simulink model "Code_for_Chp4_2DoF_LiteOfAllPlus"  (R2016b)
settings: Solver=ode4  StartTime=0  StopTime=30  FixedStep=0.0005  MaxStep=0.005  MinStep=0.001  RelTol=0.5
libraries: dspindex x2
settings Model: ExtModeTrigMode=oneshot  ExtModeArmWhenConnect=off  Creator=hp  LastModifiedBy=sfijdl
settings DataIOCC: ExternalInput=untitled.getElement(1),[],[],[],[],[],[],[],[],[],[],[],[],[],[],[],[],[],[]  SaveFormat=Array  SignalLoggingSaveFormat=ModelDataLogs  SignalLoggingName=sigsOut
settings OptimizationCC: DefaultParameterBehavior=Inlined  UseDivisionForNetSlopeComputation=on  UseFloatMulNetSlope=on  InlineInvariantSignals=on  PassReuseOutputArgsAs=Individual arguments  ExpressionDepthLimit=2147483647  ZeroExternalMemoryAtStartup=off  ZeroInternalMemoryAtStartup=off  NoFixptDivByZeroProtection=on  EfficientFloat2IntCast=on  LifeSpan=1
settings DebuggingCC: SaveWithParameterizedLinksMsg=none  UnderspecifiedInitializationDetection=Classic  MergeDetectMultiDrivingBlocksExec=none  SignalResolutionControl=TryResolveAllWithWarning  MultiTaskDSMMsg=warning  MultiTaskCondExecSysMsg=none  MultiTaskRateTransMsg=warning  ParameterTunabilityLossMsg=error  FcnCallInpInsideContextMsg=warning  StateNameClashWarn=warning  SFUnexpectedBacktrackingDiag=warning  SFNoUnconditionalDefaultTransitionDiag=warning  SFExecutionAtInitializationDiag=none
settings HardwareCC: TargetBitPerPointer=64  TargetBitPerSizeT=64  TargetBitPerPtrDiffT=64  TargetLongLongMode=on  TargetIntDivRoundTo=Zero  TargetEndianess=LittleEndian  TargetWordSize=64  TargetHWDeviceType=MATLAB Host  ProdEqTarget=off
settings ModelReferenceCC: PropagateSignalLabelsOutOfModel=off
settings RTWCC: SystemTargetFile=ert.tlc  TemplateMakefile=ert_default_tmf  Description=Embedded Coder  GenerateReport=on  IncludeHyperlinkInReport=on  LaunchReport=on  GenerateTraceInfo=on  GenerateTraceReport=on  GenerateTraceReportSl=on  GenerateTraceReportSf=on  GenerateTraceReportEml=on  GenerateCodeMetricsReport=on
settings CodeAppCC: ForceParamTrailComments=on  IgnoreCustomStorageClasses=off  MaxIdLength=128  OperatorAnnotations=on  SimulinkDataObjDesc=on  SFDataObjDesc=on  MATLABFcnDesc=on  CustomSymbolStrGlobalVar=rt$N$M  CustomSymbolStrType=$N$M  CustomSymbolStrFcn=$N$M$F  CustomSymbolStrMacro=$N$M  InsertBlockDesc=on  MATLABSourceComments=on
settings ERTTargetCC: GenerateSampleERTMain=on  CombineSignalStateStructs=on  SupportComplex=off  SupportNonInlinedSFcns=on  InlinedParameterPlacement=NonHierarchical  ERTCustomFileTemplate=example_file_process.tlc  ERTFilePackagingFormat=CompactWithDataFile
settings ConfigComp: CovMetricSettings=dw  CovHtmlReporting=on  CovSaveCumulativeToWorkspaceVar=on  CovSaveSingleToWorkspaceVar=on  CovExternalEMLEnable=off

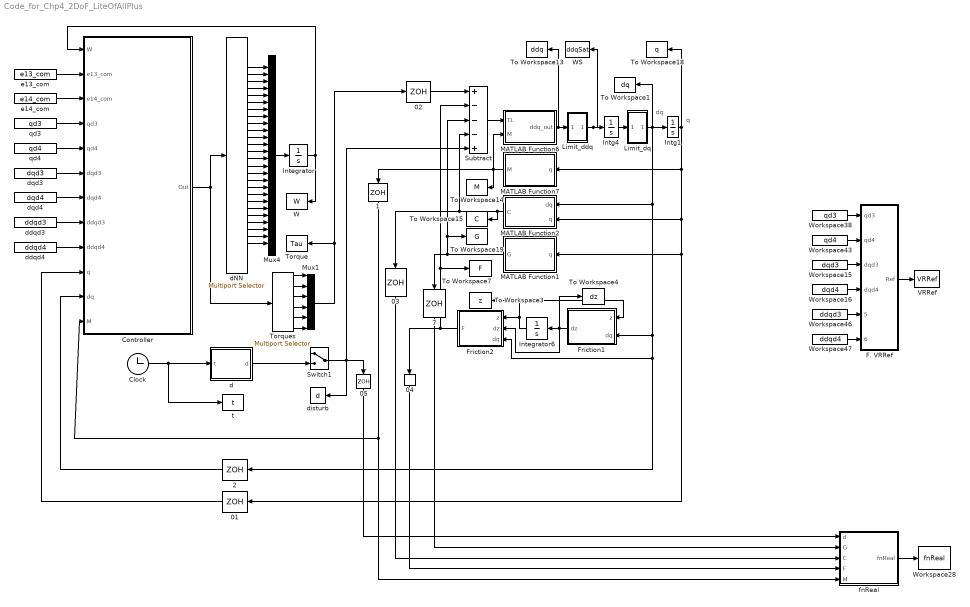
== system Code_for_Chp4_2DoF_LiteOfAllPlus ==
  note: q
  note: dq
  01 : ZeroOrderHold  SampleTime=0.0025
  02 : ZeroOrderHold  SampleTime=0.0025
  03 : ZeroOrderHold  SampleTime=0.0025
  04 : ZeroOrderHold  SampleTime=0.0025
  05 : ZeroOrderHold  SampleTime=0.0025
  1 : ZeroOrderHold  SampleTime=0.0025
  2 : ZeroOrderHold  SampleTime=0.0025
  7 : ZeroOrderHold  SampleTime=0.0025
  Clock : Clock
  Controller : MATLAB Function  TreatAsAtomicUnit=on
  F. VRRef : MATLAB Function  TreatAsAtomicUnit=on
  Friction1 : MATLAB Function  TreatAsAtomicUnit=on
  Friction2 : MATLAB Function  TreatAsAtomicUnit=on
  Integrator : Integrator  InitialCondition=[zeros(2*13,1)]
  Integrator6 : Integrator  InitialCondition=[0;0;0;0;0;0]
  Intg1 : Integrator  InitialCondition=[0.005;-0.005]
  Intg4 : Integrator  InitialCondition=[-0.1705;0.1576]
  Limit_ddq : MATLAB Function  TreatAsAtomicUnit=on
  Limit_dq : MATLAB Function  TreatAsAtomicUnit=on
  MATLAB Function1 : MATLAB Function  TreatAsAtomicUnit=on
  MATLAB Function2 : MATLAB Function  TreatAsAtomicUnit=on
  MATLAB Function6 : MATLAB Function  TreatAsAtomicUnit=on
  MATLAB Function7 : MATLAB Function  TreatAsAtomicUnit=on
  Mux1 : Mux  Inputs=6
  Mux4 : Mux  Inputs=26
  Subtract : Sum  Inputs=+---+
  Switch1 : ManualSwitch
  To Workspace1 : ToWorkspace  VariableName=dq  SampleTime=-1
  To Workspace13 : ToWorkspace  VariableName=ddq  SampleTime=-1
  To Workspace14 : ToWorkspace  VariableName=M  SampleTime=-1
  To Workspace15 : ToWorkspace  VariableName=C  SampleTime=-1
  To Workspace18 : ToWorkspace  VariableName=q  SampleTime=-1
  To Workspace19 : ToWorkspace  VariableName=G  SampleTime=-1
  To Workspace3 : ToWorkspace  VariableName=z  SampleTime=-1
  To Workspace4 : ToWorkspace  VariableName=dz  SampleTime=-1
  To Workspace7 : ToWorkspace  VariableName=F  SampleTime=-1
  Torque : ToWorkspace  VariableName=Tau  SampleTime=-1
  Torques : dspindex/Multiport Selector  rowsOrCols=Rows  idxCellArray={27,28,29,30,31,32}  idxErrMode=Clip Index
  VRRef : ToWorkspace  VariableName=VRRef  SampleTime=-1
  W : ToWorkspace  VariableName=W  SampleTime=-1
  WS : ToWorkspace  VariableName=ddqSat  SampleTime=-1
  Workspace15 : FromWorkspace  VariableName=dqd3  SampleTime=0.0025  mask(DiscretizedSource){}
      mask init:
      | %zoh
  Workspace16 : FromWorkspace  VariableName=dqd4  SampleTime=0.0025  mask(DiscretizedSource){}
      mask init:
      | %zoh
  Workspace28 : ToWorkspace  VariableName=fnReal  SampleTime=-1
  Workspace38 : FromWorkspace  VariableName=qd3  OutDataTypeStr=double  SampleTime=0.0025  mask(DiscretizedSource){}
      mask init:
      | %zoh
  Workspace43 : FromWorkspace  VariableName=qd4  SampleTime=0.0025  mask(DiscretizedSource){}
      mask init:
      | %zoh
  Workspace46 : FromWorkspace  VariableName=ddqd3  SampleTime=0.0025  mask(DiscretizedSource){}
      mask init:
      | %zoh
  Workspace47 : FromWorkspace  VariableName=ddqd4  SampleTime=0.0025  mask(DiscretizedSource){}
      mask init:
      | %zoh
  d : MATLAB Function  TreatAsAtomicUnit=on
  dNN : dspindex/Multiport Selector  rowsOrCols=Rows  idxCellArray={1,2,3,4,5,6,7,8,9,10,11,12,13,14,15,16,17,18,19,20,21,22,23,24,25,26}  idxErrMode=Clip Index
  ddqd3 : FromWorkspace  VariableName=ddqd3  SampleTime=0.0025  mask(DiscretizedSource){}
      mask init:
      | %zoh
  ddqd4 : FromWorkspace  VariableName=ddqd4  SampleTime=0.0025  mask(DiscretizedSource){}
      mask init:
      | %zoh
  disturb : ToWorkspace  VariableName=d  SampleTime=-1
  "dqd3 " : FromWorkspace  VariableName=dqd3  SampleTime=0.0025  mask(DiscretizedSource){}
      mask init:
      | %zoh
  "dqd4 " : FromWorkspace  VariableName=dqd4  SampleTime=0.0025  mask(DiscretizedSource){}
      mask init:
      | %zoh
  e13_com : FromWorkspace  VariableName=e13_com  SampleTime=0.0025  mask(DiscretizedSource){}
      mask init:
      | %zoh
  e14_com : FromWorkspace  VariableName=e14_com  SampleTime=0.0025  mask(DiscretizedSource){}
      mask init:
      | %zoh
  fnReal : MATLAB Function  TreatAsAtomicUnit=on
  qd3 : FromWorkspace  VariableName=qd3  SampleTime=0.0025  mask(DiscretizedSource){}
      mask init:
      | %zoh
  qd4 : FromWorkspace  VariableName=qd4  SampleTime=0.0025  mask(DiscretizedSource){}
      mask init:
      | %zoh
  t : ToWorkspace  VariableName=t  SampleTime=-1
  wires:
  qd3/1 -> Controller/4(qd3)
  "dqd3 "/1 -> Controller/6(dqd3)
  "dqd4 "/1 -> Controller/7(dqd4)
  ddqd3/1 -> Controller/8(ddqd3)
  ddqd4/1 -> Controller/9(ddqd4)
  MATLAB Function6/1(ddq_out) -> To Workspace13/1, Limit_ddq/1(ddq)
  MATLAB Function1/1(G) -> 7/1, To Workspace19/1, Subtract/3
  MATLAB Function2/1(C) -> To Workspace15/1, 03/1, Subtract/4
  Friction1/1(dz) -> Integrator6/1, To Workspace4/1, Friction2/2(dz)
  Integrator6/1 -> Friction1/1(z), To Workspace3/1, Friction2/1(z)
  Subtract/1 -> MATLAB Function6/1(TL)
  MATLAB Function7/1(M) -> 1/1, To Workspace14/1, MATLAB Function6/2(M)
  Intg1/1 -> 01/1, MATLAB Function1/1(q), MATLAB Function2/2(q), MATLAB Function7/1(q), To Workspace18/1
  02/1 -> Subtract/1
  Clock/1 -> t/1, d/1(t)
  7/1 -> fnReal/2(G)
  1/1 -> Controller/12(M), fnReal/5(M)
  Intg4/1 -> Limit_dq/1(dq)
  Limit_dq/1(Satdq) -> To Workspace1/1, MATLAB Function2/1(dq), 2/1, Friction2/3(dq), Friction1/2(dq), Intg1/1
  03/1 -> fnReal/3(C)
  04/1 -> fnReal/4(F)
  Switch1/1 -> 05/1, disturb/1, Subtract/5
  05/1 -> fnReal/1(d)
  fnReal/1(fnReal) -> Workspace28/1
  Limit_ddq/1(Satddq) -> WS/1, Intg4/1
  Friction2/1(F) -> 04/1, Subtract/2, To Workspace7/1
  01/1 -> Controller/10(q)
  d/1(d) -> Switch1/2
  e14_com/1 -> Controller/3(e14_com)
  e13_com/1 -> Controller/2(e13_com)
  qd4/1 -> Controller/5(qd4)
  Workspace38/1 -> F. VRRef/1(qd3)
  Workspace43/1 -> F. VRRef/2(qd4)
  Workspace47/1 -> F. VRRef/6(ddqd4)
  Workspace46/1 -> F. VRRef/5(ddqd3)
  Workspace16/1 -> F. VRRef/4(dqd4)
  Workspace15/1 -> F. VRRef/3(dqd3)
  F. VRRef/1(Ref) -> VRRef/1
  2/1 -> Controller/11(dq)
  Torques/1 -> Mux1/1
  Torques/2 -> Mux1/2
  Controller/1(Out) -> Torques/1, dNN/1
  dNN/3 -> Mux4/3
  dNN/2 -> Mux4/2
  dNN/4 -> Mux4/4
  dNN/5 -> Mux4/5
  dNN/6 -> Mux4/6
  dNN/7 -> Mux4/7
  dNN/8 -> Mux4/8
  dNN/9 -> Mux4/9
  dNN/10 -> Mux4/10
  dNN/13 -> Mux4/13
  dNN/11 -> Mux4/11
  dNN/12 -> Mux4/12
  dNN/1 -> Mux4/1
  dNN/14 -> Mux4/14
  dNN/15 -> Mux4/15
  dNN/16 -> Mux4/16
  dNN/17 -> Mux4/17
  dNN/18 -> Mux4/18
  dNN/19 -> Mux4/19
  dNN/20 -> Mux4/20
  dNN/21 -> Mux4/21
  dNN/22 -> Mux4/22
  dNN/23 -> Mux4/23
  dNN/24 -> Mux4/24
  dNN/25 -> Mux4/25
  dNN/26 -> Mux4/26
  Mux4/1 -> Integrator/1
  Integrator/1 -> W/1, Controller/1(W)
  Mux1/1 -> 02/1, Torque/1
  Torques/5 -> Mux1/5
  Torques/6 -> Mux1/6
  Torques/3 -> Mux1/3
  Torques/4 -> Mux1/4

== matlab function Code_for_Chp4_2DoF_LiteOfAllPlus/MATLAB Function1 ==
  settings: updateMethod=CONTINUOUS  sampleTime=0.0005
  data: q input; G output
function G = Gravity(q)

q3=q(1); q4=q(2);

G1 = 0; 
G2 = (817603655937935*cos(q3 + q4 + pi/2))/4611686018427387904 + (10048952709718828759483*sin(q3 + q4 + pi/2))/5764607523034234880000 + (12583885985274322167*cos(q3 + pi/2))/703687441776640000 + 10874744537588643/5070602400912917605986812821504;
G3 = (12583885985274322167*cos(q3 + pi/2))/703687441776640000 + (817603655937935*cos(q4)*cos(q3 + pi/2))/4611686018427387904 + (10048952709718828759483*cos(q4)*sin(q3 + pi/2))/5764607523034234880000 + (10048952709718828759483*cos(q3 + pi/2)*sin(q4))/5764607523034234880000 - (817603655937935*sin(q4)*sin(q3 + pi/2))/4611686018427387904;
G4 = (817603655937935*cos(q4)*cos(q3 + pi/2))/4611686018427387904 + (10048952709718828759483*cos(q4)*sin(q3 + pi/2))/5764607523034234880000 + (10048952709718828759483*cos(q3 + pi/2)*sin(q4))/5764607523034234880000 - (817603655937935*sin(q4)*sin(q3 + pi/2))/4611686018427387904;
G5 = (11873003616788183147*sin(q3 + q4 + pi/2))/230584300921369395200;
G6 = (817603655937935*cos(q3 + q4 + pi/2))/4611686018427387904 + (4927137821310187*sin(q3 + q4 + pi/2))/9223372036854775808;

G=[G1;G2;G3;G4;G5;G6]; 
end

== matlab function Code_for_Chp4_2DoF_LiteOfAllPlus/Controller ==
  settings: updateMethod=DISCRETE  sampleTime=0.0025
  data: W input; e13_com input; e14_com input; qd3 input; qd4 input; dqd3 input; dqd4 input; ddqd3 input; ddqd4 input; q input; dq input; Out output; M input
function Out = Controller(W,e13_com,e14_com,qd3,qd4,dqd3,dqd4,ddqd3,ddqd4,q,dq,M)
%% 一、参数
%     1)控制器增益
            k13=15;k14=15;    k23=2;k24=2;    k33=100;k34=100;
            K1=[k13;k14];     K2=[k23;k24];   K3=[k33;k34];
            K1=diag(K1);      K2=diag(K2);    K3=diag(K3);
%     2)双环BLF
            rho_13=.008;rho_14=.008;  rho_33=.5;rho_34=.5;
            rho_11=rho_13;rho_12=rho_14;  rho_31=rho_33;rho_32=rho_34;
%     3)RBFNN            
            nodes=13;  Tau11=60;Tau12=60;  eta1=0.01;  b=60;
            c=[-30 -25 -20 -15 -10 -5 0 5 10 15 20 25 30;
               -30 -25 -20 -15 -10 -5 0 5 10 15 20 25 30];
            
%% 二、系统输入
e1_com=[e13_com;e14_com];
qd=[qd3;qd4]; 
dqd=[dqd3;dqd4];
ddqd=[ddqd3;ddqd4];

%% 三、编码器
Delta=2*pi/2^19;
q_sample=[0;0];
for i=1:1:2
    Number=floor(q(i)/Delta)+1;
    q_sample(i)=Number*Delta;
end

%% 四、误差信号
e1=q_sample-qd;
% e1=q-(qd-.5*e1_com); % OK
de1=dq-dqd;

%% 五、虚拟控制器
miu=-K1*e1+dqd;
dmiu=-K1*de1+ddqd;

%% 六、辅助误差信号
e2=dq-miu;
e3=K2*e1+e2;

%% 七、双环BLF
%     1)外环
            u_BLF1=[e1(1)/(rho_11^2-e1(1)^2);
                    e1(2)/(rho_12^2-e1(2)^2)];     % u_BLF1：2行1列
%     2)内环
            u_BLF2_denominator_1=rho_31^2-e3(1)^2;
            u_BLF2_denominator_2=rho_32^2-e3(2)^2;
            u_BLF2=[e3(1)/u_BLF2_denominator_1;
                    e3(2)/u_BLF2_denominator_2];   % u_BLF2：2行1列
            Gain_3=diag([u_BLF2_denominator_1;u_BLF2_denominator_2]);

%% 八、RBFNN
%     1)RBF Kernel 
            xi1=[q_sample(1);dq(1)];xi2=[q_sample(2);dq(2)];
            h1=zeros(nodes,1);h2=zeros(nodes,1);
            for j=1:1:nodes
                h1(j)=exp(-norm(xi1-c(:,j))^2/(b*b));
                h2(j)=exp(-norm(xi2-c(:,j))^2/(b*b));
            end
%      2)estimate
            W1=W(1:nodes,1);W2=W(nodes+1:2*nodes,1);
            fn=[W1'*h1;W2'*h2];
%      3)dynamics of W
            dW=zeros(2*nodes,1);
            for i=1:1:nodes
                dW(i)=Tau11*h1(i)*u_BLF2(1)-eta1*W1(i); 
                dW(nodes+i)=Tau12*h2(i)*u_BLF2(2)-eta1*W2(i); 
            end

%% 九、真实控制器
%     1) 6行6列的模型矩阵
            M66 = [M(1) M(2) M(3) M(4) M(5) M(6)
                   M(7) M(8) M(9) M(10) M(11) M(12)
                   M(13) M(14) M(15) M(16) M(17) M(18)
                   M(19) M(20) M(21) M(22) M(23) M(24)
                   M(25) M(26) M(27) M(28) M(29) M(30)
                   M(31) M(32) M(33) M(34) M(35) M(36)];
%     2) 核心组件
            Torque_parts=-K2*de1-K3*e3-fn+dmiu-Gain_3*u_BLF1-diag([0.5;0.5])*u_BLF2; % Torque_parts: 2行1列
%     3) 六维输出
            Torque=M66*[0;0;Torque_parts;0;0];
% Torque_out_2=[Torque(3);Torque(4)];   

%% 十、输出
Out=[dW;Torque];  %  Torque_out_2
end

== matlab function Code_for_Chp4_2DoF_LiteOfAllPlus/MATLAB Function2 ==
  settings: updateMethod=CONTINUOUS  sampleTime=0.0005
  data: dq input; C output; q input
function C = Col(dq,q)

q3=q(1); q4=q(2); dq3=dq(1); dq4=dq(2);

C1 = (158738597992664517*dq3^2*sin(q3))/1152921504606846976 - (788574876594818524558499406425187*dq3^2*cos(q3))/93536104789177786765035829293842113257979682750464 - (31766188111850551462598880893467128091902779047347567*dq3^2*cos(q3)*cos(q4))/1532495540865888858358347027150309183618739122183602176 - (31766188111850551462598880893467128091902779047347567*dq4^2*cos(q3)*cos(q4))/1532495540865888858358347027150309183618739122183602176 + (329958928438908233217359294665525876989291241165*dq3^2*cos(q3)*sin(q4))/191561942608236107294793378393788647952342390272950272 + (329958928438908233217359294665525876989291241165*dq3^2*cos(q4)*sin(q3))/191561942608236107294793378393788647952342390272950272 + (329958928438908233217359294665525876989291241165*dq4^2*cos(q3)*sin(q4))/191561942608236107294793378393788647952342390272950272 + (329958928438908233217359294665525876989291241165*dq4^2*cos(q4)*sin(q3))/191561942608236107294793378393788647952342390272950272 + (31766188111850551462598880893467128091902779047347567*dq3^2*sin(q3)*sin(q4))/1532495540865888858358347027150309183618739122183602176 + (31766188111850551462598880893467128091902779047347567*dq4^2*sin(q3)*sin(q4))/1532495540865888858358347027150309183618739122183602176 - (31766188111850551296445381420352643978926896512304495*dq3*dq4*cos(q3)*cos(q4))/766247770432944429179173513575154591809369561091801088 + (329958928438908233217359294666797622934896747981*dq3*dq4*cos(q3)*sin(q4))/95780971304118053647396689196894323976171195136475136 + (329958928438908233217359294666797622934896747981*dq3*dq4*cos(q4)*sin(q3))/95780971304118053647396689196894323976171195136475136 + (31766188111850551296445381420352643978926896512304495*dq3*dq4*sin(q3)*sin(q4))/766247770432944429179173513575154591809369561091801088;
C2 = (9666515293019412421*dq4^2*cos(q4))/147573952589676412928 - (3932438768524053*dq4^2*sin(q4))/590295810358705651712 - (6599725983735443*dq3^2*sin(q3))/9007199254740992 - (3932438768524053*dq3*dq4*sin(q4))/295147905179352825856 + (21081034709077362555*dq3^2*cos(q3)*cos(q4))/295147905179352825856 + (21081034709077362555*dq4^2*cos(q3)*cos(q4))/295147905179352825856 - (8575983760191473*dq3^2*cos(q3)*sin(q4))/1180591620717411303424 - (8575983760191473*dq3^2*cos(q4)*sin(q3))/1180591620717411303424 - (8575983760191473*dq4^2*cos(q3)*sin(q4))/1180591620717411303424 - (8575983760191473*dq4^2*cos(q4)*sin(q3))/1180591620717411303424 - (21081034709077362555*dq3^2*sin(q3)*sin(q4))/295147905179352825856 - (21081034709077362555*dq4^2*sin(q3)*sin(q4))/295147905179352825856 + (9666515293019412421*dq3*dq4*cos(q4))/73786976294838206464 + (21081034709077362555*dq3*dq4*cos(q3)*cos(q4))/147573952589676412928 - (8575983760191473*dq3*dq4*cos(q3)*sin(q4))/590295810358705651712 - (8575983760191473*dq3*dq4*cos(q4)*sin(q3))/590295810358705651712 - (21081034709077362555*dq3*dq4*sin(q3)*sin(q4))/147573952589676412928;
C3 = (9666515293019412421*dq4^2*cos(q4))/147573952589676412928 - (3932438768524053*dq4^2*sin(q4))/590295810358705651712 - (3932438768524053*dq3*dq4*sin(q4))/295147905179352825856 + (9666515293019412421*dq3*dq4*cos(q4))/73786976294838206464;
C4 = (3932438768524053*dq3^2*sin(q4))/590295810358705651712 - (9666515293019412421*dq3^2*cos(q4))/147573952589676412928;
C5 = - (7541740619071967*dq3*dq4)/9444732965739290427392 - (7541740619071967*dq3^2)/18889465931478580854784 - (7541740619071967*dq4^2)/18889465931478580854784 - (2230692869490939*dq3^2*cos(q4))/1152921504606846976;
C6 = (3932438768524053*dq3^2*sin(q4))/590295810358705651712 + (4369139136790775*dq3*dq4)/1180591620717411303424 + (4369139136790775*dq3^2)/2361183241434822606848 + (4369139136790775*dq4^2)/2361183241434822606848 - (2962264730236869*dq3^2*cos(q4))/147573952589676412928;

C=[C1;C2;C3;C4;C5;C6]; 
end

== matlab function Code_for_Chp4_2DoF_LiteOfAllPlus/Friction1 ==
  settings: updateMethod=CONTINUOUS  sampleTime=0.0005
  data: z input; dz output; dq input
function dz = Friction1(z,dq)
 
z3=z(3); z4=z(4);   dq3=dq(1); dq4=dq(2);

dz1 = 0;
dz2 = 0;
dz3 = (32880603970571302491146779030281*dq3*atan(1000*dq3)^2)/81129638414606681695789005144064 - (13366329615528018129*dq3*z3*atan(1000*dq3))/(1801439850948198400*((6177572351796469*atan((5734161139222659*dq3*atan(1000*dq3))/90071992547409920))/144115188075855872 + 1003/2500));
dz4 = (32880603970571302491146779030281*dq4*atan(1000*dq4)^2)/81129638414606681695789005144064 - (13366329615528018129*dq4*z4*atan(1000*dq4))/(1801439850948198400*((6177572351796469*atan((5734161139222659*dq4*atan(1000*dq4))/90071992547409920))/144115188075855872 + 1003/2500));
dz5 = 0;
dz6 = 0;
dz=[dz1;dz2;dz3;dz4;dz5;dz6]; 
end

== matlab function Code_for_Chp4_2DoF_LiteOfAllPlus/Friction2 ==
  settings: updateMethod=CONTINUOUS  sampleTime=0.0005
  data: z input; dz input; F output; dq input
function F = Friction2(z,dz,dq)

z3=z(3); z4=z(4);   dz3=dz(3); dz4=dz(4);   dq3=dq(1); dq4=dq(2);

F1 = 0;
F2 = 0;
F3 = (797302866510865*dq3)/288230376151711744 + (14749*dz3)/2500 + (2331*z3)/200 - (20755908149554467968595694231197*dq3^2*atan(1000*dq3))/21267647932558653966460912964485513216;
F4 = (797302866510865*dq4)/288230376151711744 + (14749*dz4)/2500 + (2331*z4)/200 - (20755908149554467968595694231197*dq4^2*atan(1000*dq4))/21267647932558653966460912964485513216;
F4 = 1/5 * F4;
F5 = 0;
F6 = 0;
F=[F1;F2;F3;F4;F5;F6];
end

== matlab function Code_for_Chp4_2DoF_LiteOfAllPlus/MATLAB Function6 ==
  settings: updateMethod=CONTINUOUS  sampleTime=0.0005
  data: TL input; M input; ddq_out output
function ddq_out = Dynamics(TL,M)
% 姝ゅ嚱鏁颁唬琛ㄦ墽琛岋細杩炴潌閮ㄥ垎鐨勬鍔ㄥ姏瀛�
% input=[q,TL]
% output=[ddq]瑙掑姞閫熷害
% q=[1 0.2 0.2 0.2 0.2 0.2];

M66 = [M(1) M(2) M(3) M(4) M(5) M(6)
       M(7) M(8) M(9) M(10) M(11) M(12)
       M(13) M(14) M(15) M(16) M(17) M(18)
       M(19) M(20) M(21) M(22) M(23) M(24)
       M(25) M(26) M(27) M(28) M(29) M(30)
       M(31) M(32) M(33) M(34) M(35) M(36)];

ddq=M66 \ TL;  %  见纸上的公式    % ddq为6行1列

ddq_out=[ddq(3);ddq(4)];
end

== matlab function Code_for_Chp4_2DoF_LiteOfAllPlus/MATLAB Function7 ==
  settings: updateMethod=CONTINUOUS  sampleTime=0.0005
  data: q input; M output
function M = Stiffness(q)

q3=q(1);q4=q(2);

M11 = (3932438768524053*cos(q4))/590295810358705651712 - (9666515293019412421*sin(2*q3 + q4))/147573952589676412928 - (7347855351585683*cos(2*q3))/18014398509481984 - (36945533070432904259*cos(2*q3 + 2*q4))/2361183241434822606848 - (2242006792538445303*sin(2*q3 + 2*q4))/1208925819614629174706176 - (3932438768524053*cos(2*q3 + q4))/590295810358705651712 + (9666515293019412421*sin(q4))/147573952589676412928 + 6993021903434165153791/9444732965739290427392;
M12 = (1566193994333460609165*cos(q3 + q4 + pi/2))/75557863725914323419136 - (260291698974264027*sin(q3 + q4 + pi/2))/151115727451828646838272 - (158738597992664517*sin(q3 + pi/2))/1152921504606846976 - 23750155206264607/144115188075855872;
M13 = (1566193994333460609165*cos(q3 + q4 + pi/2))/75557863725914323419136 - (260291698974264027*sin(q3 + q4 + pi/2))/151115727451828646838272 - (158738597992664517*sin(q3 + pi/2))/1152921504606846976;
M14 = (1566193994333460609165*cos(q3 + q4 + pi/2))/75557863725914323419136 - (260291698974264027*sin(q3 + q4 + pi/2))/151115727451828646838272;
M15 = - (3951197109736239241155*cos(q3 + q4 + pi/2))/75557863725914323419136 - (2242006792538445279*sin(q3 + q4 + pi/2))/1208925819614629174706176 - (3932438768524053*cos(q3 + pi/2))/590295810358705651712 - 2364964252341131/5316911983139663491615228241121378304;
M16 = (392149993849384621*cos(q3 + q4 + pi/2))/75557863725914323419136 - (260291698974264035*sin(q3 + q4 + pi/2))/151115727451828646838272;
M22 = (6599725983735443*cos(q3))/4503599627370496 + (3932438768524053*cos(q4))/295147905179352825856 + (9666515293019412421*sin(q4))/73786976294838206464 + (8575983760191473*cos(q3)*cos(q4))/590295810358705651712 + (21081034709077362555*cos(q3)*sin(q4))/147573952589676412928 + (21081034709077362555*cos(q4)*sin(q3))/147573952589676412928 - (8575983760191473*sin(q3)*sin(q4))/590295810358705651712 + 802526512685661487937/295147905179352825856;
M23 = (6599725983735443*cos(q3))/9007199254740992 + (3932438768524053*cos(q4))/295147905179352825856 + (9666515293019412421*sin(q4))/73786976294838206464 + (8575983760191473*cos(q3)*cos(q4))/1180591620717411303424 + (21081034709077362555*cos(q3)*sin(q4))/295147905179352825856 + (21081034709077362555*cos(q4)*sin(q3))/295147905179352825856 - (8575983760191473*sin(q3)*sin(q4))/1180591620717411303424 + 292870962545184539457/295147905179352825856;
M24 = (3932438768524053*cos(q4))/590295810358705651712 + (9666515293019412421*sin(q4))/147573952589676412928 + (8575983760191473*cos(q3)*cos(q4))/1180591620717411303424 + (21081034709077362555*cos(q3)*sin(q4))/295147905179352825856 + (21081034709077362555*cos(q4)*sin(q3))/295147905179352825856 - (8575983760191473*sin(q3)*sin(q4))/1180591620717411303424 + 36296309188291035969/295147905179352825856;
M25 = (2230692869490939*sin(q4))/1152921504606846976 + (304047738388393*cos(q3)*sin(q4))/144115188075855872 + (304047738388393*cos(q4)*sin(q3))/144115188075855872 + 315508820003156273/2361183241434822606848;
M26 = (3932438768524053*cos(q4))/590295810358705651712 + (2962264730236869*sin(q4))/147573952589676412928 + (8575983760191473*cos(q3)*cos(q4))/1180591620717411303424 + (6460198293038971*cos(q3)*sin(q4))/295147905179352825856 + (6460198293038971*cos(q4)*sin(q3))/295147905179352825856 - (8575983760191473*sin(q3)*sin(q4))/1180591620717411303424 + 29720514162674078529/590295810358705651712;
M33 = (3932438768524053*cos(q4))/295147905179352825856 + (9666515293019412421*sin(q4))/73786976294838206464 + 292870962545184539457/295147905179352825856;
M34 = (3932438768524053*cos(q4))/590295810358705651712 + (9666515293019412421*sin(q4))/147573952589676412928 + 36296309188291035969/295147905179352825856;
M35 = (2230692869490939*sin(q4))/1152921504606846976 + 315508820003156273/2361183241434822606848;
M36 = (3932438768524053*cos(q4))/590295810358705651712 + (2962264730236869*sin(q4))/147573952589676412928 + 29720514162674078529/590295810358705651712;
M44 = 0.1230;
M45 = 1.3362e-04;
M46 = 0.0503;
M55 = 0.0529;
M56 = 1.2030e-06;
M66 = 0.0503;

M = [M11; M12; M13; M14; M15; M16;
     M12; M22; M23; M24; M25; M26;   
     M13; M23; M33; M34; M35; M36;   
     M14; M24; M34; M44; M45; M46;   
     M15; M25; M35; M45; M55; M56;   
     M16; M26; M36; M46; M56; M66;];
end

== matlab function Code_for_Chp4_2DoF_LiteOfAllPlus/Limit_dq ==
  settings: updateMethod=CONTINUOUS
  data: dq input; Satdq output
function Satdq = Satdq(dq)
dqMax=3;
% dqMax=inf;   [0;0;-0.0853;0.0849;0;0]  [0;0;-0.1705;0.1576;0;0]  [0;0;-0.12;0.1;0;0]
for i=1:1:2
    if dq(i)>dqMax
        dq(i)=dqMax;
    elseif dq(i)<-dqMax
        dq(i)=-dqMax;
    end
end
Satdq=[dq(1);dq(2)];
end

== matlab function Code_for_Chp4_2DoF_LiteOfAllPlus/F. VRRef ==
  settings: updateMethod=CONTINUOUS  sampleTime=0.0025
  data: qd3 input; qd4 input; dqd3 input; dqd4 input; ddqd3 input; ddqd4 input; Ref output
function Ref = RefTT(qd3,qd4,dqd3,dqd4,ddqd3,ddqd4)
Ref=[qd3;qd4;dqd3;dqd4;ddqd3;ddqd4]; 
end

== matlab function Code_for_Chp4_2DoF_LiteOfAllPlus/Limit_ddq ==
  settings: updateMethod=CONTINUOUS
  data: ddq input; Satddq output
function Satddq = Satddq(ddq)
Amax=pi/2;
Amax=pi;
for i=1:1:2
    if ddq(i)>Amax
        ddq(i)=Amax;
    elseif ddq(i)<-Amax
        ddq(i)=-Amax;
    end
end
Satddq=[ddq(1);ddq(2)];
end

== matlab function Code_for_Chp4_2DoF_LiteOfAllPlus/fnReal ==
  settings: updateMethod=DISCRETE  sampleTime=0.0025
  data: d input; G input; C input; F input; M input; fnReal output
function fnReal = fnReal(d,G,C,F,M)
M66 = [M(1) M(2) M(3) M(4) M(5) M(6)
       M(7) M(8) M(9) M(10) M(11) M(12)
       M(13) M(14) M(15) M(16) M(17) M(18)
       M(19) M(20) M(21) M(22) M(23) M(24)
       M(25) M(26) M(27) M(28) M(29) M(30)
       M(31) M(32) M(33) M(34) M(35) M(36)];
fnReal1=inv(M66)*(d-C-F-G);
fnReal2=.5*inv(M66)*(-G);
fnReal=[fnReal1;fnReal2];
end

== matlab function Code_for_Chp4_2DoF_LiteOfAllPlus/d ==
  settings: updateMethod=CONTINUOUS  sampleTime=0.0005
  data: d output; t input
function d = disturb(t)
% d=0.1*rand(6,1);
% d=0.1*rand(6,1)*3*sin(0.5*t);
if t>15 && t<21.2
% 仅HyOFC可以
%     d=[120.0*sin(1*(t-15));
%                          0;
%        100.0*sin(1*(t-15));
%                zeros(3,1)];
% M-BC和HyOFC都可以          
    d=[50.0*sin(1*(t-15));
                         0;
       15.0*sin(1*(t-15));
               zeros(3,1)];
else
    d=zeros(6,1);
end
end
